simulink model "specificTaskTemplate"  (R2012b)
settings: Solver=FixedStepDiscrete  StartTime=0.0  StopTime=10.0  FixedStep=0.001  RelTol=1e-3
undefined symbols (not defined in the file): acquireMethods, clickPercentage, clickRefractoryPeriod, cuedText, cuedTextLength, cumulativeDwell, cursorDiameter, cursorDownColor, cursorNeuralColor, cursorNonneuralColor, displayShape, displayShape_1, displayShape_10, displayShape_2, displayShape_3, displayShape_4, displayShape_5, displayShape_6, displayShape_7, displayShape_8, displayShape_9, dwellRefractoryPeriod, gain, gloveBias, gloveLPDenominator, gloveLPNumerator, height, height_1, height_10, height_2, height_3, height_4, height_5, height_6, height_7, height_8, height_9, holdTime, ID, ID_1, ID_10, ID_2, ID_3, ID_4, ID_5, ID_6, ID_7, ID_8, ID_9, initialInput, initialLockout, initialState, inputType, keyboard, keyboardDims, keyPressedTime, maxTaskTime, mouseLPDenominator, mouseLPNumerator, mouseOffset ... (+122)
(part 1 of 2)
settings Model: Creator=gilja  LastModifiedBy=NPTL
settings SolverCC: EnableConcurrentExecution=on  ConcurrentTasks=on
settings DataIOCC: SaveOutput=off  SignalLogging=off  SaveTime=off
settings OptimizationCC: InlineParams=on  InlineInvariantSignals=on  EnhancedBackFolding=on  EfficientFloat2IntCast=on  SimCompilerOptimization=On
settings DebuggingCC: UnderspecifiedInitializationDetection=Simplified
settings HardwareCC: ProdIntDivRoundTo=Zero  ProdEndianess=LittleEndian  ProdHWDeviceType=Generic->32-bit x86 compatible
settings RTWCC: SystemTargetFile=xpctarget.tlc  TemplateMakefile=xpc_default_tmf  Description=xPC Target  ProcessScript=xpctarget_make_rtw_hook  RTWCompilerOptimization=On
settings CodeAppCC: MaxIdLength=62
settings xpcTargetCC: TargetFcnLib=ansi_tfl_table_tmw.mat  CodeReplacementLibrary=XPC_BLAS  ParMdlRefBuildCompliant=on  ConcurrentExecutionCompliant=on  CombineSignalStateStructs=off  GRTInterface=on  xPCTaskExecutionProfile=on  xPCRL32EventNumber=5000  xPCisDownloadable=off  xPCLoadParamSetFile=off  xPCConcurrentTasks=off  xPCEnableSFAnimation=off

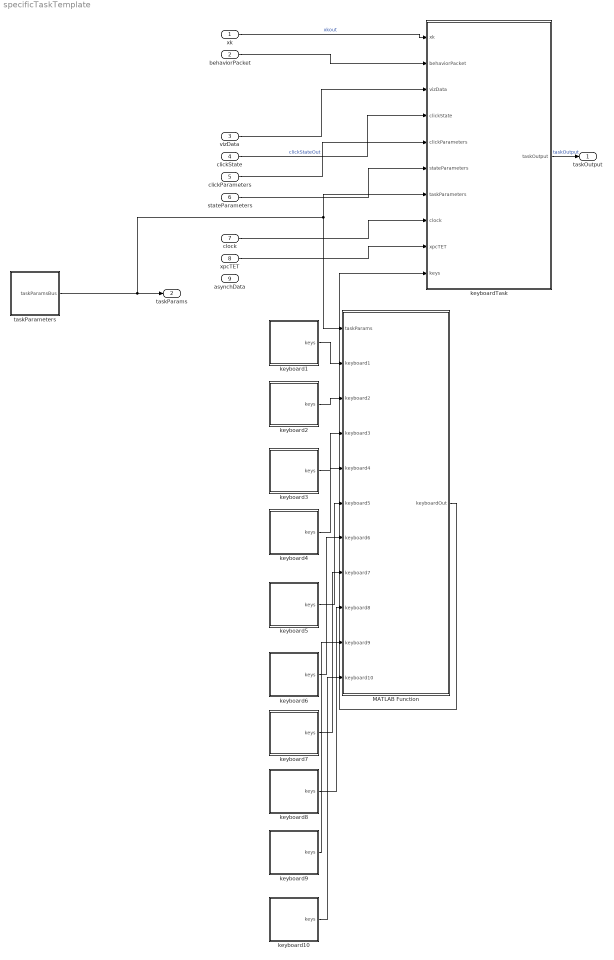
== system specificTaskTemplate ==
  xk : Inport  OutDataTypeStr=double  PortDimensions=[5 1]  SampleTime=[0.001,0]
  behaviorPacket : Inport  Port=2  OutDataTypeStr=Bus: behaviorPacketBus  SampleTime=[0.001,0]
  vizData : Inport  Port=3  OutDataTypeStr=Bus: peripheralData  SampleTime=[0.001,0]
  clickState : Inport  Port=4  OutDataTypeStr=uint16  PortDimensions=1  SampleTime=[0.001,0]
  clickParameters : Inport  Port=5  OutDataTypeStr=Bus: clickParametersBus  SampleTime=[0.001,0]
  stateParameters : Inport  Port=6  OutDataTypeStr=Bus: stateParams  SampleTime=[0.001,0]
  clock : Inport  Port=7  OutDataTypeStr=uint32  PortDimensions=1  SampleTime=[0.001,0]
  xpcTET : Inport  Port=8  OutDataTypeStr=double  PortDimensions=1  SampleTime=[0.001,0]
  asynchData : Inport  Port=9  OutDataTypeStr=Bus: peripheralData  SampleTime=[0.001,0]
  MATLAB Function : MATLAB Function  TreatAsAtomicUnit=on
  keyboard1 : Subsystem
  keyboard10 : Subsystem
  keyboard2 : Subsystem
  keyboard3 : Subsystem
  keyboard4 : Subsystem
  keyboard5 : Subsystem
  keyboard6 : Subsystem
  keyboard7 : Subsystem
  keyboard8 : Subsystem
  keyboard9 : Subsystem
  keyboardTask : MATLAB Function  TreatAsAtomicUnit=on
  taskParameters : Subsystem
  taskOutput : Outport  OutDataTypeStr=Bus: taskOutput  PortDimensions=1  SampleTime=[0.001,0]  BusOutputAsStruct=on
  taskParams : Outport  Port=2  OutDataTypeStr=Bus: taskParamsBus  SampleTime=[0.001,0]
  wires:
  xk/1 -> keyboardTask/1(xk)  "xkout"
  behaviorPacket/1 -> keyboardTask/2(behaviorPacket)
  vizData/1 -> keyboardTask/3(vizData)
  clickState/1 -> keyboardTask/4(clickState)  "clickStateOut"
  clickParameters/1 -> keyboardTask/5(clickParameters)
  clock/1 -> keyboardTask/8(clock)
  xpcTET/1 -> keyboardTask/9(xpcTET)
  keyboardTask/1(taskOutput) -> taskOutput/1  "taskOutput"
  stateParameters/1 -> keyboardTask/6(stateParameters)
  taskParameters/1(taskParamsBus) -> taskParams/1, MATLAB Function/1(taskParams), keyboardTask/7(taskParameters)
  keyboard1/1(keys) -> MATLAB Function/2(keyboard1)
  keyboard2/1(keys) -> MATLAB Function/3(keyboard2)
  MATLAB Function/1(keyboardOut) -> keyboardTask/10(keys)
  keyboard3/1(keys) -> MATLAB Function/4(keyboard3)
  keyboard4/1(keys) -> MATLAB Function/5(keyboard4)
  keyboard5/1(keys) -> MATLAB Function/6(keyboard5)
  keyboard6/1(keys) -> MATLAB Function/7(keyboard6)
  keyboard7/1(keys) -> MATLAB Function/8(keyboard7)
  keyboard8/1(keys) -> MATLAB Function/9(keyboard8)
  keyboard9/1(keys) -> MATLAB Function/10(keyboard9)
  keyboard10/1(keys) -> MATLAB Function/11(keyboard10)

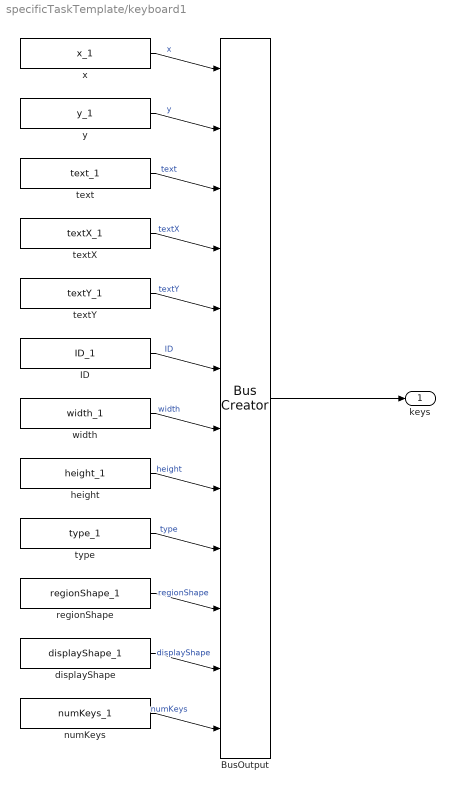
== system specificTaskTemplate/keyboard1 ==
  BusOutput : BusCreator  Inputs=x,y,text,textX,textY,ID,width,height,type,regionShape,displayShape,numKeys  OutDataTypeStr=Bus: keysParamsBus
  ID : Constant  Value=ID_1
  displayShape : Constant  Value=displayShape_1
  height : Constant  Value=height_1
  numKeys : Constant  Value=numKeys_1
  regionShape : Constant  Value=regionShape_1
  text : Constant  Value=text_1
  textX : Constant  Value=textX_1
  textY : Constant  Value=textY_1
  type : Constant  Value=type_1
  width : Constant  Value=width_1
  x : Constant  Value=x_1
  y : Constant  Value=y_1
  keys : Outport
  wires:
  x/1 -> BusOutput/1  "x"
  y/1 -> BusOutput/2  "y"
  text/1 -> BusOutput/3  "text"
  textX/1 -> BusOutput/4  "textX"
  textY/1 -> BusOutput/5  "textY"
  ID/1 -> BusOutput/6  "ID"
  width/1 -> BusOutput/7  "width"
  height/1 -> BusOutput/8  "height"
  type/1 -> BusOutput/9  "type"
  regionShape/1 -> BusOutput/10  "regionShape"
  displayShape/1 -> BusOutput/11  "displayShape"
  numKeys/1 -> BusOutput/12  "numKeys"
  BusOutput/1 -> keys/1

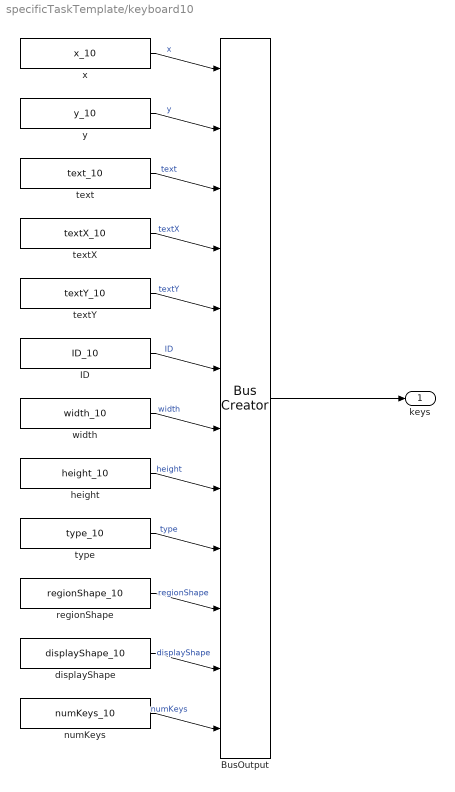
== system specificTaskTemplate/keyboard10 ==
  BusOutput : BusCreator  Inputs=x,y,text,textX,textY,ID,width,height,type,regionShape,displayShape,numKeys  OutDataTypeStr=Bus: keysParamsBus
  ID : Constant  Value=ID_10
  displayShape : Constant  Value=displayShape_10
  height : Constant  Value=height_10
  numKeys : Constant  Value=numKeys_10
  regionShape : Constant  Value=regionShape_10
  text : Constant  Value=text_10
  textX : Constant  Value=textX_10
  textY : Constant  Value=textY_10
  type : Constant  Value=type_10
  width : Constant  Value=width_10
  x : Constant  Value=x_10
  y : Constant  Value=y_10
  keys : Outport  OutDataTypeStr=Bus: keysParamsBus
  wires:
  x/1 -> BusOutput/1  "x"
  y/1 -> BusOutput/2  "y"
  text/1 -> BusOutput/3  "text"
  textX/1 -> BusOutput/4  "textX"
  textY/1 -> BusOutput/5  "textY"
  ID/1 -> BusOutput/6  "ID"
  width/1 -> BusOutput/7  "width"
  height/1 -> BusOutput/8  "height"
  type/1 -> BusOutput/9  "type"
  regionShape/1 -> BusOutput/10  "regionShape"
  displayShape/1 -> BusOutput/11  "displayShape"
  numKeys/1 -> BusOutput/12  "numKeys"
  BusOutput/1 -> keys/1

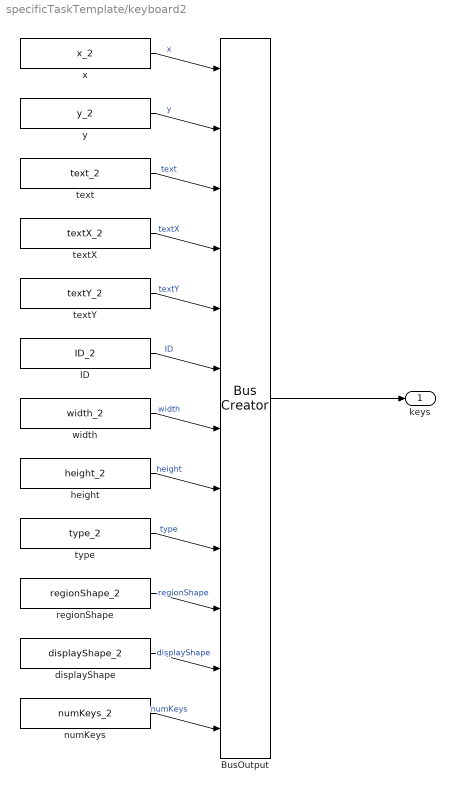
== system specificTaskTemplate/keyboard2 ==
  BusOutput : BusCreator  Inputs=x,y,text,textX,textY,ID,width,height,type,regionShape,displayShape,numKeys  OutDataTypeStr=Bus: keysParamsBus
  ID : Constant  Value=ID_2
  displayShape : Constant  Value=displayShape_2
  height : Constant  Value=height_2
  numKeys : Constant  Value=numKeys_2
  regionShape : Constant  Value=regionShape_2
  text : Constant  Value=text_2
  textX : Constant  Value=textX_2
  textY : Constant  Value=textY_2
  type : Constant  Value=type_2
  width : Constant  Value=width_2
  x : Constant  Value=x_2
  y : Constant  Value=y_2
  keys : Outport  OutDataTypeStr=Bus: keysParamsBus
  wires:
  x/1 -> BusOutput/1  "x"
  y/1 -> BusOutput/2  "y"
  text/1 -> BusOutput/3  "text"
  textX/1 -> BusOutput/4  "textX"
  textY/1 -> BusOutput/5  "textY"
  ID/1 -> BusOutput/6  "ID"
  width/1 -> BusOutput/7  "width"
  height/1 -> BusOutput/8  "height"
  type/1 -> BusOutput/9  "type"
  regionShape/1 -> BusOutput/10  "regionShape"
  displayShape/1 -> BusOutput/11  "displayShape"
  numKeys/1 -> BusOutput/12  "numKeys"
  BusOutput/1 -> keys/1

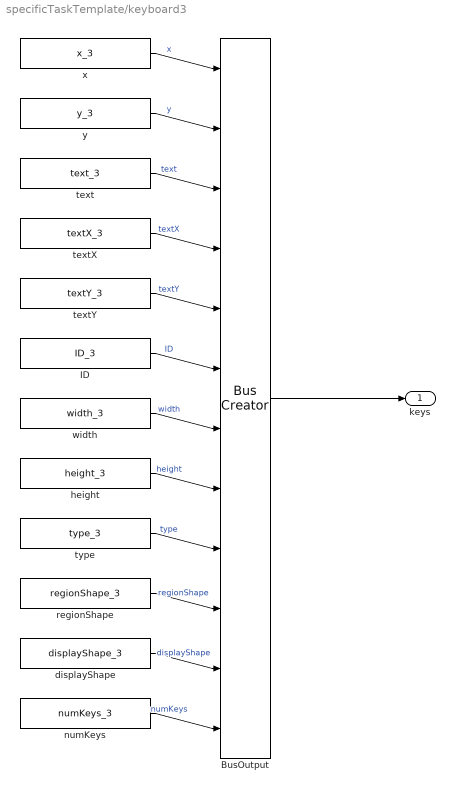
== system specificTaskTemplate/keyboard3 ==
  BusOutput : BusCreator  Inputs=x,y,text,textX,textY,ID,width,height,type,regionShape,displayShape,numKeys  OutDataTypeStr=Bus: keysParamsBus
  ID : Constant  Value=ID_3
  displayShape : Constant  Value=displayShape_3
  height : Constant  Value=height_3
  numKeys : Constant  Value=numKeys_3
  regionShape : Constant  Value=regionShape_3
  text : Constant  Value=text_3
  textX : Constant  Value=textX_3
  textY : Constant  Value=textY_3
  type : Constant  Value=type_3
  width : Constant  Value=width_3
  x : Constant  Value=x_3
  y : Constant  Value=y_3
  keys : Outport  OutDataTypeStr=Bus: keysParamsBus
  wires:
  x/1 -> BusOutput/1  "x"
  y/1 -> BusOutput/2  "y"
  text/1 -> BusOutput/3  "text"
  textX/1 -> BusOutput/4  "textX"
  textY/1 -> BusOutput/5  "textY"
  ID/1 -> BusOutput/6  "ID"
  width/1 -> BusOutput/7  "width"
  height/1 -> BusOutput/8  "height"
  type/1 -> BusOutput/9  "type"
  regionShape/1 -> BusOutput/10  "regionShape"
  displayShape/1 -> BusOutput/11  "displayShape"
  numKeys/1 -> BusOutput/12  "numKeys"
  BusOutput/1 -> keys/1

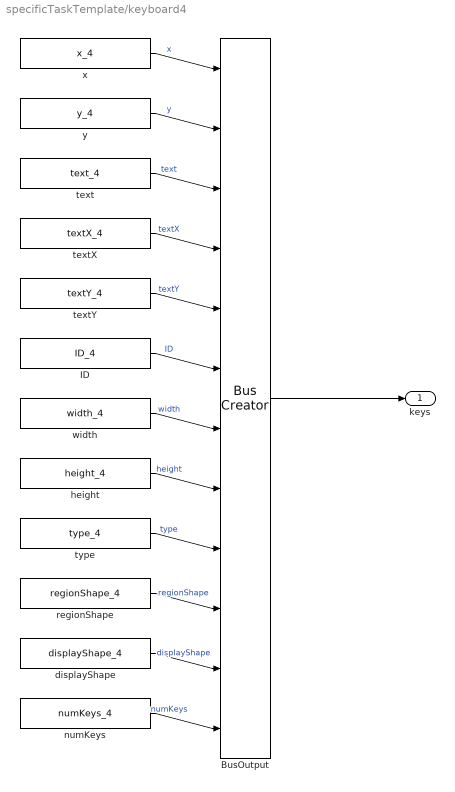
== system specificTaskTemplate/keyboard4 ==
  BusOutput : BusCreator  Inputs=x,y,text,textX,textY,ID,width,height,type,regionShape,displayShape,numKeys  OutDataTypeStr=Bus: keysParamsBus
  ID : Constant  Value=ID_4
  displayShape : Constant  Value=displayShape_4
  height : Constant  Value=height_4
  numKeys : Constant  Value=numKeys_4
  regionShape : Constant  Value=regionShape_4
  text : Constant  Value=text_4
  textX : Constant  Value=textX_4
  textY : Constant  Value=textY_4
  type : Constant  Value=type_4
  width : Constant  Value=width_4
  x : Constant  Value=x_4
  y : Constant  Value=y_4
  keys : Outport  OutDataTypeStr=Bus: keysParamsBus
  wires:
  x/1 -> BusOutput/1  "x"
  y/1 -> BusOutput/2  "y"
  text/1 -> BusOutput/3  "text"
  textX/1 -> BusOutput/4  "textX"
  textY/1 -> BusOutput/5  "textY"
  ID/1 -> BusOutput/6  "ID"
  width/1 -> BusOutput/7  "width"
  height/1 -> BusOutput/8  "height"
  type/1 -> BusOutput/9  "type"
  regionShape/1 -> BusOutput/10  "regionShape"
  displayShape/1 -> BusOutput/11  "displayShape"
  numKeys/1 -> BusOutput/12  "numKeys"
  BusOutput/1 -> keys/1

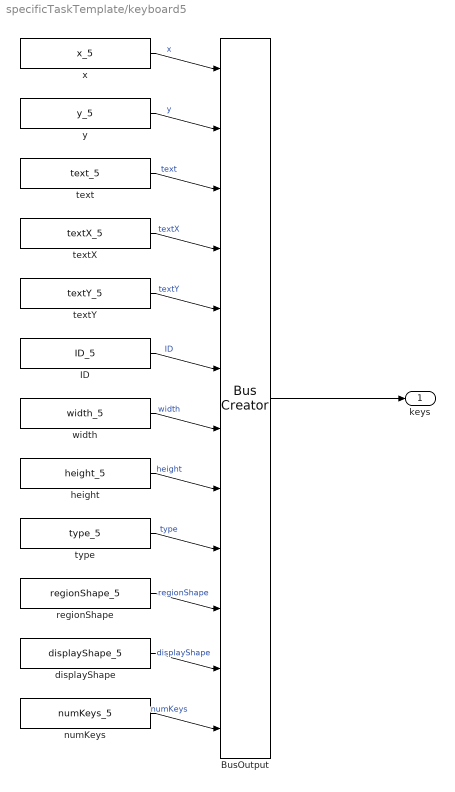
== system specificTaskTemplate/keyboard5 ==
  BusOutput : BusCreator  Inputs=x,y,text,textX,textY,ID,width,height,type,regionShape,displayShape,numKeys  OutDataTypeStr=Bus: keysParamsBus
  ID : Constant  Value=ID_5
  displayShape : Constant  Value=displayShape_5
  height : Constant  Value=height_5
  numKeys : Constant  Value=numKeys_5
  regionShape : Constant  Value=regionShape_5
  text : Constant  Value=text_5
  textX : Constant  Value=textX_5
  textY : Constant  Value=textY_5
  type : Constant  Value=type_5
  width : Constant  Value=width_5
  x : Constant  Value=x_5
  y : Constant  Value=y_5
  keys : Outport  OutDataTypeStr=Bus: keysParamsBus
  wires:
  x/1 -> BusOutput/1  "x"
  y/1 -> BusOutput/2  "y"
  text/1 -> BusOutput/3  "text"
  textX/1 -> BusOutput/4  "textX"
  textY/1 -> BusOutput/5  "textY"
  ID/1 -> BusOutput/6  "ID"
  width/1 -> BusOutput/7  "width"
  height/1 -> BusOutput/8  "height"
  type/1 -> BusOutput/9  "type"
  regionShape/1 -> BusOutput/10  "regionShape"
  displayShape/1 -> BusOutput/11  "displayShape"
  numKeys/1 -> BusOutput/12  "numKeys"
  BusOutput/1 -> keys/1

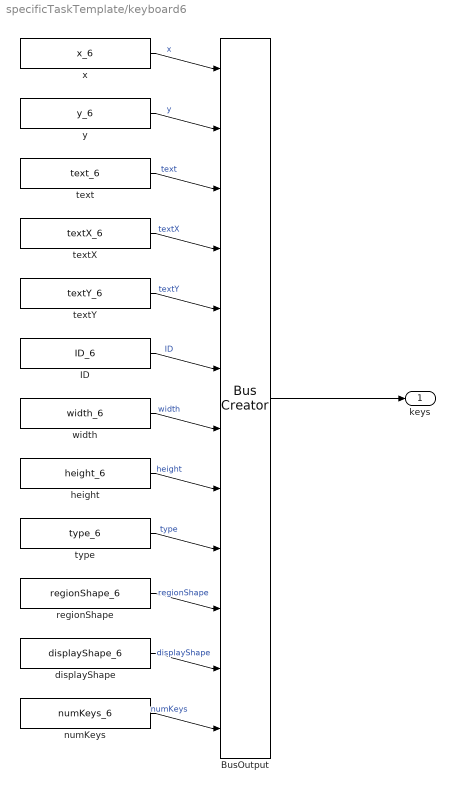
== system specificTaskTemplate/keyboard6 ==
  BusOutput : BusCreator  Inputs=x,y,text,textX,textY,ID,width,height,type,regionShape,displayShape,numKeys  OutDataTypeStr=Bus: keysParamsBus
  ID : Constant  Value=ID_6
  displayShape : Constant  Value=displayShape_6
  height : Constant  Value=height_6
  numKeys : Constant  Value=numKeys_6
  regionShape : Constant  Value=regionShape_6
  text : Constant  Value=text_6
  textX : Constant  Value=textX_6
  textY : Constant  Value=textY_6
  type : Constant  Value=type_6
  width : Constant  Value=width_6
  x : Constant  Value=x_6
  y : Constant  Value=y_6
  keys : Outport  OutDataTypeStr=Bus: keysParamsBus
  wires:
  x/1 -> BusOutput/1  "x"
  y/1 -> BusOutput/2  "y"
  text/1 -> BusOutput/3  "text"
  textX/1 -> BusOutput/4  "textX"
  textY/1 -> BusOutput/5  "textY"
  ID/1 -> BusOutput/6  "ID"
  width/1 -> BusOutput/7  "width"
  height/1 -> BusOutput/8  "height"
  type/1 -> BusOutput/9  "type"
  regionShape/1 -> BusOutput/10  "regionShape"
  displayShape/1 -> BusOutput/11  "displayShape"
  numKeys/1 -> BusOutput/12  "numKeys"
  BusOutput/1 -> keys/1

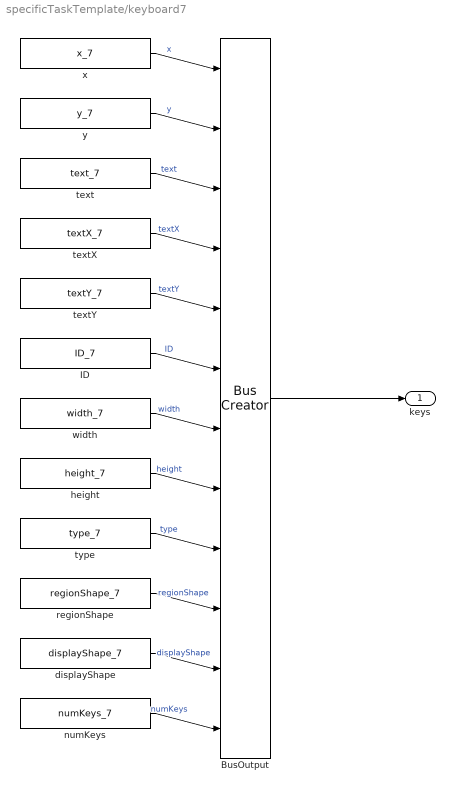
== system specificTaskTemplate/keyboard7 ==
  BusOutput : BusCreator  Inputs=x,y,text,textX,textY,ID,width,height,type,regionShape,displayShape,numKeys  OutDataTypeStr=Bus: keysParamsBus
  ID : Constant  Value=ID_7
  displayShape : Constant  Value=displayShape_7
  height : Constant  Value=height_7
  numKeys : Constant  Value=numKeys_7
  regionShape : Constant  Value=regionShape_7
  text : Constant  Value=text_7
  textX : Constant  Value=textX_7
  textY : Constant  Value=textY_7
  type : Constant  Value=type_7
  width : Constant  Value=width_7
  x : Constant  Value=x_7
  y : Constant  Value=y_7
  keys : Outport  OutDataTypeStr=Bus: keysParamsBus
  wires:
  x/1 -> BusOutput/1  "x"
  y/1 -> BusOutput/2  "y"
  text/1 -> BusOutput/3  "text"
  textX/1 -> BusOutput/4  "textX"
  textY/1 -> BusOutput/5  "textY"
  ID/1 -> BusOutput/6  "ID"
  width/1 -> BusOutput/7  "width"
  height/1 -> BusOutput/8  "height"
  type/1 -> BusOutput/9  "type"
  regionShape/1 -> BusOutput/10  "regionShape"
  displayShape/1 -> BusOutput/11  "displayShape"
  numKeys/1 -> BusOutput/12  "numKeys"
  BusOutput/1 -> keys/1

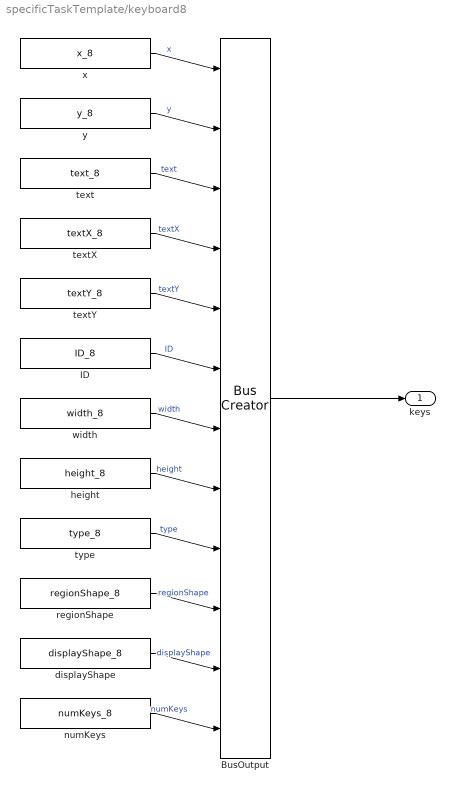
== system specificTaskTemplate/keyboard8 ==
  BusOutput : BusCreator  Inputs=x,y,text,textX,textY,ID,width,height,type,regionShape,displayShape,numKeys  OutDataTypeStr=Bus: keysParamsBus
  ID : Constant  Value=ID_8
  displayShape : Constant  Value=displayShape_8
  height : Constant  Value=height_8
  numKeys : Constant  Value=numKeys_8
  regionShape : Constant  Value=regionShape_8
  text : Constant  Value=text_8
  textX : Constant  Value=textX_8
  textY : Constant  Value=textY_8
  type : Constant  Value=type_8
  width : Constant  Value=width_8
  x : Constant  Value=x_8
  y : Constant  Value=y_8
  keys : Outport  OutDataTypeStr=Bus: keysParamsBus
  wires:
  x/1 -> BusOutput/1  "x"
  y/1 -> BusOutput/2  "y"
  text/1 -> BusOutput/3  "text"
  textX/1 -> BusOutput/4  "textX"
  textY/1 -> BusOutput/5  "textY"
  ID/1 -> BusOutput/6  "ID"
  width/1 -> BusOutput/7  "width"
  height/1 -> BusOutput/8  "height"
  type/1 -> BusOutput/9  "type"
  regionShape/1 -> BusOutput/10  "regionShape"
  displayShape/1 -> BusOutput/11  "displayShape"
  numKeys/1 -> BusOutput/12  "numKeys"
  BusOutput/1 -> keys/1

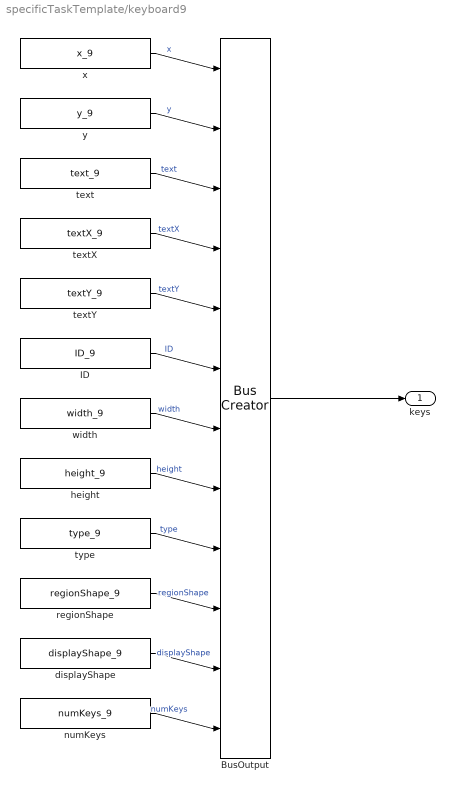
== system specificTaskTemplate/keyboard9 ==
  BusOutput : BusCreator  Inputs=x,y,text,textX,textY,ID,width,height,type,regionShape,displayShape,numKeys  OutDataTypeStr=Bus: keysParamsBus
  ID : Constant  Value=ID_9
  displayShape : Constant  Value=displayShape_9
  height : Constant  Value=height_9
  numKeys : Constant  Value=numKeys_9
  regionShape : Constant  Value=regionShape_9
  text : Constant  Value=text_9
  textX : Constant  Value=textX_9
  textY : Constant  Value=textY_9
  type : Constant  Value=type_9
  width : Constant  Value=width_9
  x : Constant  Value=x_9
  y : Constant  Value=y_9
  keys : Outport  OutDataTypeStr=Bus: keysParamsBus
  wires:
  x/1 -> BusOutput/1  "x"
  y/1 -> BusOutput/2  "y"
  text/1 -> BusOutput/3  "text"
  textX/1 -> BusOutput/4  "textX"
  textY/1 -> BusOutput/5  "textY"
  ID/1 -> BusOutput/6  "ID"
  width/1 -> BusOutput/7  "width"
  height/1 -> BusOutput/8  "height"
  type/1 -> BusOutput/9  "type"
  regionShape/1 -> BusOutput/10  "regionShape"
  displayShape/1 -> BusOutput/11  "displayShape"
  numKeys/1 -> BusOutput/12  "numKeys"
  BusOutput/1 -> keys/1

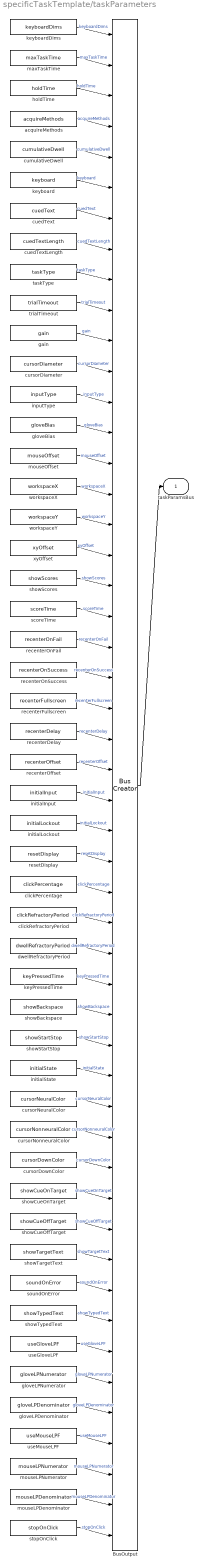
== system specificTaskTemplate/taskParameters ==
  BusOutput : BusCreator  Inputs=keyboardDims,maxTaskTime,holdTime,acquireMethods,cumulativeDwell,keyboard,cuedText,cuedTextLength,taskType,trialTimeout,gain,cursorDiameter,inputType,gloveBias,mouseOffset,workspaceX,workspaceY,xyOffset,showScores,scoreTime,recenterOnFail,recenterOnSuccess,recenterFullscreen,recenterDelay,recenterOffset,initialInput,initialLockout,resetDisplay,clickPercentage,clickRefractoryPeriod,dwellRefractoryPeriod,keyPressedTime,showBackspace,showStartStop,initialState,cursorNeuralColor,cursorNonneuralColor,cursorDownColor,showCueOnTarget,showCueOffTarget,showTargetText,soundOnError,showTypedText,useGloveLPF,gloveLPNumerator,gloveLPDenominator,useMouseLPF,mouseLPNumerator,mouseLPDenominator,stopOnClick  OutDataTypeStr=Bus: taskParamsBus
  acquireMethods : Constant  Value=acquireMethods
  clickPercentage : Constant  Value=clickPercentage
  clickRefractoryPeriod : Constant  Value=clickRefractoryPeriod
  cuedText : Constant  Value=cuedText
  cuedTextLength : Constant  Value=cuedTextLength
  cumulativeDwell : Constant  Value=cumulativeDwell
  cursorDiameter : Constant  Value=cursorDiameter
  cursorDownColor : Constant  Value=cursorDownColor
  cursorNeuralColor : Constant  Value=cursorNeuralColor
  cursorNonneuralColor : Constant  Value=cursorNonneuralColor
  dwellRefractoryPeriod : Constant  Value=dwellRefractoryPeriod
  gain : Constant  Value=gain
  gloveBias : Constant  Value=gloveBias
  gloveLPDenominator : Constant  Value=gloveLPDenominator
  gloveLPNumerator : Constant  Value=gloveLPNumerator
  holdTime : Constant  Value=holdTime
  initialInput : Constant  Value=initialInput
  initialLockout : Constant  Value=initialLockout
  initialState : Constant  Value=initialState
  inputType : Constant  Value=inputType
  keyPressedTime : Constant  Value=keyPressedTime
  keyboard : Constant  Value=keyboard
  keyboardDims : Constant  Value=keyboardDims
  maxTaskTime : Constant  Value=maxTaskTime
  mouseLPDenominator : Constant  Value=mouseLPDenominator
  mouseLPNumerator : Constant  Value=mouseLPNumerator
  mouseOffset : Constant  Value=mouseOffset
  recenterDelay : Constant  Value=recenterDelay
  recenterFullscreen : Constant  Value=recenterFullscreen
  recenterOffset : Constant  Value=recenterOffset
  recenterOnFail : Constant  Value=recenterOnFail
  recenterOnSuccess : Constant  Value=recenterOnSuccess
  resetDisplay : Constant  Value=resetDisplay
  scoreTime : Constant  Value=scoreTime
  showBackspace : Constant  Value=showBackspace
  showCueOffTarget : Constant  Value=showCueOffTarget
  showCueOnTarget : Constant  Value=showCueOnTarget
  showScores : Constant  Value=showScores
  showStartStop : Constant  Value=showStartStop
  showTargetText : Constant  Value=showTargetText
  showTypedText : Constant  Value=showTypedText
  soundOnError : Constant  Value=soundOnError
  stopOnClick : Constant  Value=stopOnClick
  taskType : Constant  Value=taskType
  trialTimeout : Constant  Value=trialTimeout
  useGloveLPF : Constant  Value=useGloveLPF
  useMouseLPF : Constant  Value=useMouseLPF
  workspaceX : Constant  Value=workspaceX
  workspaceY : Constant  Value=workspaceY
  xyOffset : Constant  Value=xyOffset
  taskParamsBus : Outport
  wires:
  BusOutput/1 -> taskParamsBus/1
  stopOnClick/1 -> BusOutput/50  "stopOnClick"
  mouseLPDenominator/1 -> BusOutput/49  "mouseLPDenominator"
  mouseLPNumerator/1 -> BusOutput/48  "mouseLPNumerator"
  useMouseLPF/1 -> BusOutput/47  "useMouseLPF"
  gloveLPDenominator/1 -> BusOutput/46  "gloveLPDenominator"
  gloveLPNumerator/1 -> BusOutput/45  "gloveLPNumerator"
  useGloveLPF/1 -> BusOutput/44  "useGloveLPF"
  showTypedText/1 -> BusOutput/43  "showTypedText"
  soundOnError/1 -> BusOutput/42  "soundOnError"
  showTargetText/1 -> BusOutput/41  "showTargetText"
  showCueOffTarget/1 -> BusOutput/40  "showCueOffTarget"
  showCueOnTarget/1 -> BusOutput/39  "showCueOnTarget"
  cursorDownColor/1 -> BusOutput/38  "cursorDownColor"
  cursorNonneuralColor/1 -> BusOutput/37  "cursorNonneuralColor"
  cursorNeuralColor/1 -> BusOutput/36  "cursorNeuralColor"
  initialState/1 -> BusOutput/35  "initialState"
  showStartStop/1 -> BusOutput/34  "showStartStop"
  showBackspace/1 -> BusOutput/33  "showBackspace"
  keyPressedTime/1 -> BusOutput/32  "keyPressedTime"
  dwellRefractoryPeriod/1 -> BusOutput/31  "dwellRefractoryPeriod"
  clickRefractoryPeriod/1 -> BusOutput/30  "clickRefractoryPeriod"
  clickPercentage/1 -> BusOutput/29  "clickPercentage"
  resetDisplay/1 -> BusOutput/28  "resetDisplay"
  initialLockout/1 -> BusOutput/27  "initialLockout"
  initialInput/1 -> BusOutput/26  "initialInput"
  recenterOffset/1 -> BusOutput/25  "recenterOffset"
  recenterDelay/1 -> BusOutput/24  "recenterDelay"
  recenterFullscreen/1 -> BusOutput/23  "recenterFullscreen"
  recenterOnSuccess/1 -> BusOutput/22  "recenterOnSuccess"
  recenterOnFail/1 -> BusOutput/21  "recenterOnFail"
  scoreTime/1 -> BusOutput/20  "scoreTime"
  showScores/1 -> BusOutput/19  "showScores"
  xyOffset/1 -> BusOutput/18  "xyOffset"
  workspaceY/1 -> BusOutput/17  "workspaceY"
  workspaceX/1 -> BusOutput/16  "workspaceX"
  mouseOffset/1 -> BusOutput/15  "mouseOffset"
  gloveBias/1 -> BusOutput/14  "gloveBias"
  inputType/1 -> BusOutput/13  "inputType"
  cursorDiameter/1 -> BusOutput/12  "cursorDiameter"
  gain/1 -> BusOutput/11  "gain"
  trialTimeout/1 -> BusOutput/10  "trialTimeout"
  taskType/1 -> BusOutput/9  "taskType"
  cuedTextLength/1 -> BusOutput/8  "cuedTextLength"
  cuedText/1 -> BusOutput/7  "cuedText"
  keyboard/1 -> BusOutput/6  "keyboard"
  cumulativeDwell/1 -> BusOutput/5  "cumulativeDwell"
  acquireMethods/1 -> BusOutput/4  "acquireMethods"
  holdTime/1 -> BusOutput/3  "holdTime"
  maxTaskTime/1 -> BusOutput/2  "maxTaskTime"
  keyboardDims/1 -> BusOutput/1  "keyboardDims"

== matlab function specificTaskTemplate/MATLAB Function ==
  data: taskParams input; keyboardOut output Bus: keysParamsBus; keyboard1 input Bus: keysParamsBus; keyboard2 input Bus: keysParamsBus; keyboard3 input; keyboard4 input; keyboard5 input; keyboard6 input; keyboard7 input; keyboard8 input; keyboard9 input; keyboard10 input
function keyboardOut = chooseKeyboard(taskParams, keyboard1, keyboard2, keyboard3, keyboard4, keyboard5, keyboard6, keyboard7, keyboard8, keyboard9, keyboard10)
%#codegen

switch taskParams.keyboard
    case uint16(keyboardConstants.KEYBOARD_QWERTY1)
        keyboardOut = keyboard1;
        
    case uint16(keyboardConstants.KEYBOARD_QWERTY2)
        keyboardOut = keyboard2;
        
    case uint16(keyboardConstants.KEYBOARD_GRID_6X6)
        keyboardOut = keyboard3;
        
    case uint16(keyboardConstants.KEYBOARD_GRID_7X7)
        keyboardOut = keyboard4;
        
    case uint16(keyboardConstants.KEYBOARD_GRID_8X8)
        keyboardOut = keyboard5;
        
    case uint16(keyboardConstants.KEYBOARD_GRID_9X9)
        keyboardOut = keyboard6;

    case uint16(keyboardConstants.KEYBOARD_GRID_10X10)
        keyboardOut = keyboard7;
    
    case uint16(keyboardConstants.KEYBOARD_QABCD)
        keyboardOut = keyboard8;

    case uint16(keyboardConstants.KEYBOARD_OPTIII)
        keyboardOut = keyboard9;

    case uint16(keyboardConstants.KEYBOARD_GRID_5X5)
        keyboardOut = keyboard10;
        
    otherwise
        keyboardOut = keyboard1;
end
